simulink model "Test3Part2"  (R2024a)
settings: Solver=VariableStepAuto  StartTime=0.0  StopTime=1000  RelTol=1e-3
libraries: simulink_extras x4, matrix_library x4
settings Model: Creator=katutu  LastModifiedBy=katutu

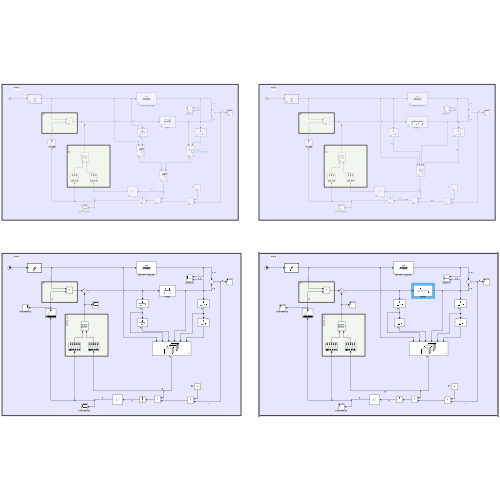
[thumbnail: Simulink's stored preview of the top-level diagram]
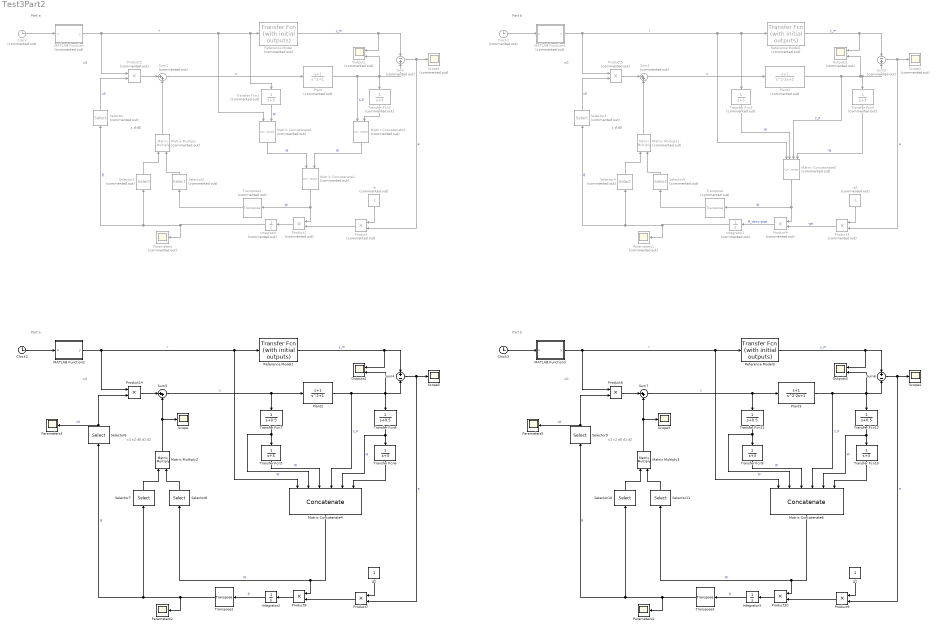
== system Test3Part2 ==
  note: Part a
  note: c
      | d
      | d0
  note: c0
  note: c
      | d
      | d0
  note: c0
  note: Part b
  note: Part a
  note: c1
      | c2
      | d0
      | d1
      | d2
  note: c0
  note: c1
      | c2
      | d0
      | d1
      | d2
  note: Part b
  note: c0
  -g : Constant  Commented=on  Value=-1
  -g1 : Constant  Commented=on  Value=-1
  Clock : Clock  Commented=on
  Clock1 : Clock  Commented=on
  Clock2 : Clock
  Clock3 : Clock
  Integrator : Integrator  Commented=on
  Integrator1 : Integrator  Commented=on
  Integrator2 : Integrator
  Integrator3 : Integrator
  MATLAB Function : MATLAB Function  Commented=on  TreatAsAtomicUnit=on
  MATLAB Function1 : MATLAB Function  Commented=on  TreatAsAtomicUnit=on
  MATLAB Function2 : MATLAB Function  TreatAsAtomicUnit=on
  MATLAB Function3 : MATLAB Function  TreatAsAtomicUnit=on
  Matrix Concatenate1 : Concatenate  Commented=on  Mode=Multidimensional array  ConcatenateDimension=2
  Matrix Concatenate2 : Concatenate  Commented=on  Mode=Multidimensional array  ConcatenateDimension=2
  Matrix Concatenate3 : Concatenate  Commented=on  Mode=Multidimensional array  ConcatenateDimension=2
  Matrix Concatenate4 : Concatenate  NumInputs=6  Mode=Multidimensional array
  Matrix Concatenate5 : Concatenate  Commented=on  NumInputs=4  Mode=Multidimensional array  ConcatenateDimension=2
  Matrix Concatenate6 : Concatenate  NumInputs=6  Mode=Multidimensional array
  Matrix Multiply : Product  Commented=on  Multiplication=Matrix(*)
  Matrix Multiply1 : Product  Commented=on  Multiplication=Matrix(*)
  Matrix Multiply2 : Product  Multiplication=Matrix(*)
  Matrix Multiply3 : Product  Multiplication=Matrix(*)
  Outputs : Scope  Commented=on  NumInputPorts=2
  Outputs1 : Scope  Commented=on  NumInputPorts=2
  Outputs2 : Scope  NumInputPorts=2
  Outputs3 : Scope  NumInputPorts=2
  Parameters : Scope  Commented=on
  Parameters1 : Scope  Commented=on
  Parameters{2..5} (4 alike) : Scope
  Plant : TransferFcn  Commented=on  Numerator=[1 1]  Denominator=[1 0 1]
  Plant1 : TransferFcn  Commented=on  Numerator=[1 1]  Denominator=[1 -2 1]
  Plant2 : TransferFcn  Numerator=[1 1]  Denominator=[1 0 1]
  Plant3 : TransferFcn  Numerator=[1 1]  Denominator=[1 -2 1]
  Product{,1..5} (6 alike) : Product  Commented=on
  Product{6..10,14} (6 alike) : Product
  Reference Model : simulink_extras/Additional Linear/Transfer Fcn (with initial outputs)  Commented=on  N=[1 3]  D="[1  6 5]"  Y0=0  U0=0
  Reference Model1 : simulink_extras/Additional Linear/Transfer Fcn (with initial outputs)  Commented=on  N=[1 3]  D="[1  6 5]"  Y0=0  U0=0
  Reference Model2 : simulink_extras/Additional Linear/Transfer Fcn (with initial outputs)  N=[1 3]  D="[1  6 5]"  Y0=0  U0=0
  Reference Model3 : simulink_extras/Additional Linear/Transfer Fcn (with initial outputs)  N=[1 3]  D="[1  6 5]"  Y0=0  U0=0
  Scope{,3..5} (4 alike) : Scope
  Scope1 : Scope  Commented=on
  Scope2 : Scope  Commented=on
  Selector : Selector  Commented=on  InputPortWidth=4  IndexOptions=Index vector (dialog)  Indices=[1]  OutputSizes=1
  Selector{1..2,4..5} (4 alike) : Selector  Commented=on  InputPortWidth=4  IndexOptions=Index vector (dialog)  Indices=[2 3 4]  OutputSizes=1
  Selector{7..8,10..11} (4 alike) : Selector  InputPortWidth=6  IndexOptions=Index vector (dialog)  Indices=[2 3 4 5 6]  OutputSizes=1
  Selector3 : Selector  Commented=on  InputPortWidth=4  IndexOptions=Index vector (dialog)  Indices=[1]  OutputSizes=1
  Selector6 : Selector  InputPortWidth=6  IndexOptions=Index vector (dialog)  Indices=[1]  OutputSizes=1
  Selector9 : Selector  InputPortWidth=6  IndexOptions=Index vector (dialog)  Indices=[1]  OutputSizes=1
  Sum : Sum  Commented=on  Inputs=-|+
  Sum1 : Sum  Commented=on  Inputs=|++
  Sum2 : Sum  Commented=on  Inputs=-|+
  Sum3 : Sum  Commented=on  Inputs=|++
  Sum4 : Sum  Inputs=+|-
  Sum5 : Sum  Inputs=|++
  Sum6 : Sum  Inputs=+|-
  Sum7 : Sum  Inputs=|++
  Transfer Fcn{1..4} (4 alike) : TransferFcn  Commented=on  Denominator=[1 3]
  Transfer Fcn{5..6,9..10} (4 alike) : TransferFcn  Denominator=[1 3]
  Transfer Fcn{7..8,11..12} (4 alike) : TransferFcn  Denominator=[1 0.5]
  Transpose : matrix_library/Transpose  Commented=on
  Transpose1 : matrix_library/Transpose  Commented=on
  Transpose2 : matrix_library/Transpose
  Transpose3 : matrix_library/Transpose
  g1 : Constant
  g2 : Constant
  wires:
  Reference Model/1 -> Outputs/1, Sum/1  "y_m"
  Sum/1 -> Product/2, Scope1/1  "e"
  -g/1 -> Product/1
  Clock/1 -> MATLAB Function/1(u)
  Product1/1 -> Integrator/1
  Matrix Concatenate2/1 -> Product1/1, Transpose1/1  "W"
  Plant/1 -> Matrix Concatenate3/1, Transfer Fcn2/1, Sum/2, Outputs/2  "y_p"
  Matrix Concatenate3/1 -> Matrix Concatenate2/2  "W"
  Transfer Fcn2/1 -> Matrix Concatenate3/2
  Product/1 -> Product1/2
  MATLAB Function/1(y) -> Product2/1, Transfer Fcn1/1, Reference Model/1, Matrix Concatenate1/1  "r"
  Sum1/1 -> Plant/1  "u"
  Transfer Fcn1/1 -> Matrix Concatenate1/2  "W"
  Matrix Concatenate1/1 -> Matrix Concatenate2/1  "W"
  Selector/1 -> Product2/2  "c0"
  Product2/1 -> Sum1/1
  Selector1/1 -> Matrix Multiply/1
  Matrix Multiply/1 -> Sum1/2
  Selector2/1 -> Matrix Multiply/2
  Integrator/1 -> Parameters/1, Selector/1, Selector1/1  "θ"
  Matrix Concatenate5/1 -> Transpose/1, Product4/1  "W"
  MATLAB Function1/1(y) -> Product5/1, Reference Model1/1, Transfer Fcn3/1, Matrix Concatenate5/1  "r"
  Transfer Fcn3/1 -> Matrix Concatenate5/2  "W"
  Matrix Multiply1/1 -> Sum3/2
  Plant1/1 -> Matrix Concatenate5/3, Transfer Fcn4/1, Sum2/2, Outputs1/2  "y_p"
  Product5/1 -> Sum3/1
  Transfer Fcn4/1 -> Matrix Concatenate5/4  "W"
  Selector5/1 -> Matrix Multiply1/2
  Reference Model1/1 -> Outputs1/1, Sum2/1  "y_m"
  -g1/1 -> Product3/1
  Product4/1 -> Integrator1/1  "θ_dot=-gwe"
  Sum2/1 -> Scope2/1, Product3/2  "e"
  Selector4/1 -> Matrix Multiply1/1
  Integrator1/1 -> Parameters1/1, Selector4/1, Selector3/1  "θ"
  Clock1/1 -> MATLAB Function1/1(u)
  Selector3/1 -> Product5/2  "c0"
  Sum3/1 -> Plant1/1  "u"
  Product3/1 -> Product4/2  "-ge"
  Transpose1/1 -> Selector2/1
  Transpose/1 -> Selector5/1
  Product7/1 -> Product8/2
  Clock2/1 -> MATLAB Function2/1(u)
  Sum4/1 -> Product7/2, Scope5/1  "e"
  Matrix Concatenate4/1 -> Selector8/1, Product8/1  "W"
  Selector6/1 -> Product14/2, Parameters3/1  "c0"
  Sum5/1 -> Plant2/1, Transfer Fcn7/1  "u"
  MATLAB Function2/1(y) -> Product14/1, Reference Model2/1, Matrix Concatenate4/1  "r"
  Reference Model2/1 -> Outputs2/1, Sum4/1  "y_m"
  Plant2/1 -> Matrix Concatenate4/4, Outputs2/2, Transfer Fcn8/1, Sum4/2  "y_p"
  g2/1 -> Product7/1
  Product8/1 -> Integrator2/1
  Selector7/1 -> Matrix Multiply2/1
  Integrator2/1 -> Transpose2/1  "θ"
  Transfer Fcn6/1 -> Matrix Concatenate4/6
  Transfer Fcn5/1 -> Matrix Concatenate4/3  "W"
  Selector8/1 -> Matrix Multiply2/2
  Product14/1 -> Sum5/1
  Transfer Fcn7/1 -> Transfer Fcn5/1, Matrix Concatenate4/2  "W"
  Transfer Fcn8/1 -> Matrix Concatenate4/5, Transfer Fcn6/1  "W"
  Matrix Multiply2/1 -> Sum5/2, Scope/1
  Transpose2/1 -> Selector7/1, Selector6/1, Parameters2/1  "θ"
  Selector10/1 -> Matrix Multiply3/1
  Transfer Fcn10/1 -> Matrix Concatenate6/6
  Product6/1 -> Sum7/1
  Plant3/1 -> Matrix Concatenate6/4, Outputs3/2, Transfer Fcn12/1, Sum6/2  "y_p"
  g1/1 -> Product9/1
  Sum7/1 -> Plant3/1, Transfer Fcn11/1  "u"
  Product10/1 -> Integrator3/1
  Transpose3/1 -> Selector10/1, Selector9/1, Parameters4/1  "θ"
  Selector11/1 -> Matrix Multiply3/2
  MATLAB Function3/1(y) -> Product6/1, Reference Model3/1, Matrix Concatenate6/1  "r"
  Sum6/1 -> Product9/2, Scope4/1  "e"
  Selector9/1 -> Product6/2, Parameters5/1  "c0"
  Transfer Fcn11/1 -> Transfer Fcn9/1, Matrix Concatenate6/2  "W"
  Reference Model3/1 -> Outputs3/1, Sum6/1  "y_m"
  Matrix Multiply3/1 -> Sum7/2, Scope3/1
  Transfer Fcn9/1 -> Matrix Concatenate6/3  "W"
  Matrix Concatenate6/1 -> Selector11/1, Product10/1  "W"
  Clock3/1 -> MATLAB Function3/1(u)
  Product9/1 -> Product10/2
  Integrator3/1 -> Transpose3/1  "θ"
  Transfer Fcn12/1 -> Matrix Concatenate6/5, Transfer Fcn10/1  "W"

== matlab function Test3Part2/MATLAB Function ==
  data: u input; y output
function y = fcn(u)

y = 2*sin(u);

== matlab function Test3Part2/MATLAB Function2 ==
  data: u input; y output
function y = fcn(u)

y = 2*sin(u);

== matlab function Test3Part2/MATLAB Function3 ==
  data: u input; y output
function y = fcn(u)

y = 2*sin(u);

== matlab function Test3Part2/MATLAB Function1 ==
  data: u input; y output
function y = fcn(u)

y = 2*sin(u);
